simulink model "main_model"  (R2022a)
settings: Solver=FixedStepDiscrete  StartTime=0.0  StopTime=10.0  FixedStep=1/CLK_FREQ  RelTol=1e-3
undefined symbols (not defined in the file): CLK_FREQ, FLTR_PERIOD
settings Model: DataDictionary=mainDictionary.sldd  Creator=andre  LastModifiedBy=andre

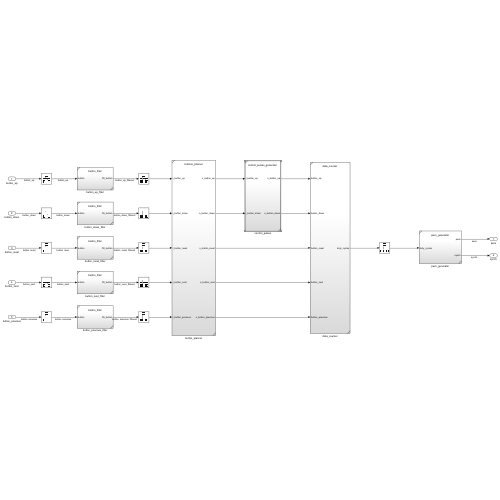
[thumbnail: Simulink's stored preview of the top-level diagram]
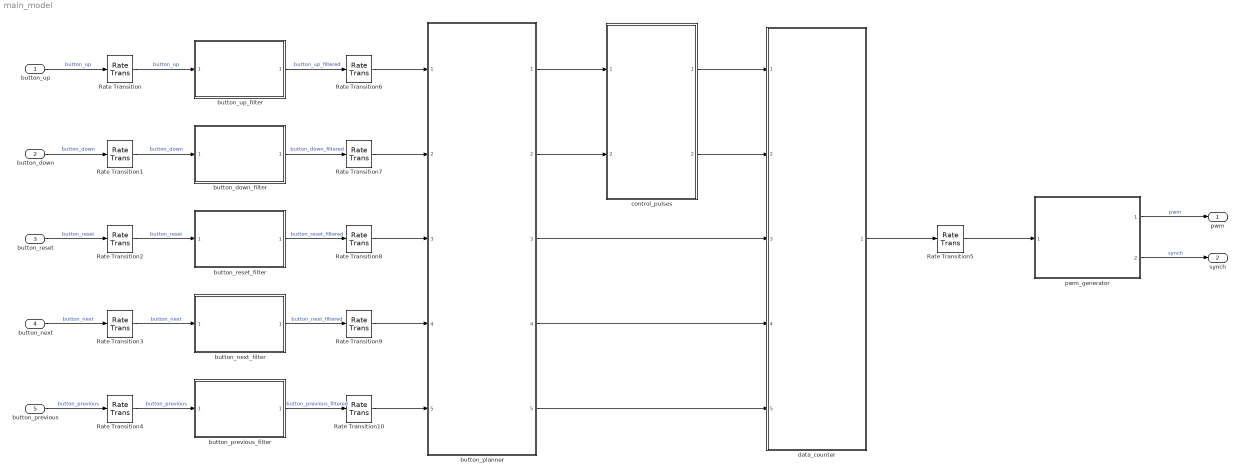
== system main_model ==
  button_up : Inport  OutDataTypeStr=boolean  PortDimensions=1
  button_down : Inport  Port=2  OutDataTypeStr=boolean  PortDimensions=1
  button_reset : Inport  Port=3  OutDataTypeStr=boolean  PortDimensions=1
  button_next : Inport  Port=4  OutDataTypeStr=boolean  PortDimensions=1
  button_previous : Inport  Port=5  OutDataTypeStr=boolean  PortDimensions=1
  Rate Transition{,1..4} (5 alike) : RateTransition  OutPortSampleTime=round(FLTR_PERIOD*CLK_FREQ/(2e9))/CLK_FREQ
  Rate Transition{6..10} (5 alike) : RateTransition  OutPortSampleTime=1/CLK_FREQ
  Rate Transition5 : RateTransition  OutPortSampleTime=3.9e-7
  button_down_filter : Subsystem  ReferencedSubsystem=button_filter
  button_next_filter : Subsystem  ReferencedSubsystem=button_filter
  button_planner : Subsystem  ReferencedSubsystem=buttons_planner
  button_previous_filter : Subsystem  ReferencedSubsystem=button_filter
  button_reset_filter : Subsystem  ReferencedSubsystem=button_filter
  button_up_filter : Subsystem  ReferencedSubsystem=button_filter
  control_pulses : Subsystem  ReferencedSubsystem=control_pulses_generator
  data_counter : Subsystem  ReferencedSubsystem=data_counter
  pwm_generator : Subsystem  ReferencedSubsystem=pwm_generator
  pwm : Outport  OutDataTypeStr=boolean  PortDimensions=3
  synch : Outport  Port=2  OutDataTypeStr=boolean  PortDimensions=1
  wires:
  Rate Transition/1 -> button_up_filter/1  "button_up"
  Rate Transition1/1 -> button_down_filter/1  "button_down"
  Rate Transition2/1 -> button_reset_filter/1  "button_reset"
  Rate Transition3/1 -> button_next_filter/1  "button_next"
  Rate Transition4/1 -> button_previous_filter/1  "button_previous"
  button_up/1 -> Rate Transition/1  "button_up"
  button_down/1 -> Rate Transition1/1  "button_down"
  button_reset/1 -> Rate Transition2/1  "button_reset"
  button_next/1 -> Rate Transition3/1  "button_next"
  button_previous/1 -> Rate Transition4/1  "button_previous"
  button_up_filter/1 -> Rate Transition6/1  "button_up_filtered"
  button_down_filter/1 -> Rate Transition7/1  "button_down_filtered"
  button_reset_filter/1 -> Rate Transition8/1  "button_reset_filtered"
  button_next_filter/1 -> Rate Transition9/1  "button_next_filtered"
  button_previous_filter/1 -> Rate Transition10/1  "button_previous_filtered"
  control_pulses/2 -> data_counter/2
  control_pulses/1 -> data_counter/1
  data_counter/1 -> Rate Transition5/1
  Rate Transition5/1 -> pwm_generator/1
  pwm_generator/1 -> pwm/1  "pwm"
  pwm_generator/2 -> synch/1  "synch"
  Rate Transition10/1 -> button_planner/5
  Rate Transition6/1 -> button_planner/1
  Rate Transition7/1 -> button_planner/2
  Rate Transition8/1 -> button_planner/3
  Rate Transition9/1 -> button_planner/4
  button_planner/1 -> control_pulses/1
  button_planner/2 -> control_pulses/2
  button_planner/3 -> data_counter/3
  button_planner/4 -> data_counter/4
  button_planner/5 -> data_counter/5
